simulink model "RoboBlock"  (R2020a)
settings: Solver=ode45  StartTime=0.0  StopTime=inf  FixedStep=0.050  RelTol=1e-3
model workspace (MAT data in the model file):
  Sig = Simulink.Signal
  Sig.DataType = 'auto'
  Sig.Dimensions = -1
  Sig.DimensionsMode = 'auto'
  Sig.Complexity = 'auto'
  Sig.SampleTime = -1
  Sig.SamplingMode = 'auto'
  Var = 0
libraries: simulink x2, dspmathops x1, fuzblock x1
settings Model: PauseTimes=7  Creator=user  LastModifiedBy=hjcam
settings DataIOCC: LimitDataPoints=on  SaveFormat=Array  ReturnWorkspaceOutputs=off
settings OptimizationCC: BlockReduction=off  BooleanDataType=off  LifeSpan=inf
settings DebuggingCC: SaveWithParameterizedLinksMsg=none  UnderspecifiedInitializationDetection=Classic  MergeDetectMultiDrivingBlocksExec=none  SignalResolutionControl=TryResolveAllWithWarning  SFUnexpectedBacktrackingDiag=warning  SFNoUnconditionalDefaultTransitionDiag=warning  SFExecutionAtInitializationDiag=none  ArithmeticOperatorsInVariantConditions=warning
settings HardwareCC: ProdBitPerPointer=32  ProdBitPerSizeT=32  ProdBitPerPtrDiffT=32  ProdLargestAtomicFloat=None  ProdIntDivRoundTo=Undefined  ProdEndianess=Unspecified  ProdWordSize=32  ProdHWDeviceType=32-bit Generic  TargetBitPerPointer=64  TargetBitPerSizeT=64  TargetBitPerPtrDiffT=64  TargetLongLongMode=on  TargetIntDivRoundTo=Zero  TargetEndianess=LittleEndian  TargetWordSize=64  TargetHWDeviceType=MATLAB Host  ProdEqTarget=off
settings ModelReferenceCC: PropagateSignalLabelsOutOfModel=off
settings SFSimCC: SimUseLocalCustomCode=off  CustomCodeUndefinedFunction=UseInterfaceOnly
settings RTWCC: RTWUseLocalCustomCode=off
settings CodeAppCC: StateflowObjectComments=on
settings GRTTargetCC: TargetLangStandard=C89/C90 (ANSI)
settings ConfigComp: CovMetricSettings=dw  CovHtmlReporting=on  CovSaveCumulativeToWorkspaceVar=on  CovSaveSingleToWorkspaceVar=on  CovExternalEMLEnable=off  CovSFcnEnable=off

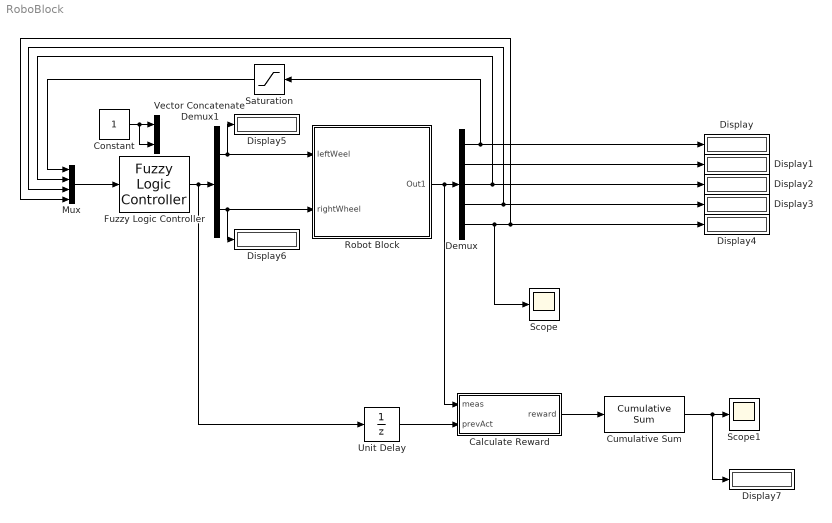
== system RoboBlock ==
  Calculate Reward : Subsystem
  Constant : Constant  VectorParams1D=off
  Cumulative Sum : dspmathops/Cumulative Sum  dim=Channels (running sum)  InputProcessing=Columns as channels (frame based)  reset_popup=None  roundingMode=Floor  overflowMode=off  outputDataTypeStr=Inherit: Same as accumulator  outputMin=[]  outputMax=[]  outputLastDataTypeStr=Inherit: Same as accumulator
  Demux : Demux  Outputs=5
  Demux1 : Demux  Outputs=2
  Display{,1..7} (8 alike) : Display
  Fuzzy Logic Controller : fuzblock/Fuzzy Logic  Controller  FIS=robot  OutputSampleNumber=101  DataType=double  FuzzifiedInputs=off  RuleFiringStrengths=off  RuleOutputs=off  AggregatedOutputs=off  SimulateUsing=Interpreted execution  OutOfRangeInputValueMessage=warning  NoRuleFiredMessage=warning  EmptyOutputFuzzySetMessage=warning
  Mux : Mux
  Robot Block : Subsystem  mask(Two-wheel Mobile Robot Model){stID=5013501, modeVal=off, initAngle=-0.628, simStep=0.050, Xpos=2.2597, Ypos=5.1629, isDemo=off}
      mask prompts: stID "Please Enter your UOW student number"; modeVal "Velocity Measurement Mode, select this to disable animations and to allow for the measurement of the velocity of the robot"; initAngle "Set the starting angle (Radians)"; simStep "Override Simulation Step (Defualt is 0.01)"; Xpos "(X,Y)"
      mask help:
      | Robot: Two-wheel robot is driven by two parallel wheels; the speed of each wheel could be set separately
      | Target: target is a single moving point in 2D space
      | Obstacle: obstacle is a group of polygons.
      | Block inputs:
      | vl : velocity of left wheel
      | vr : velocity of right wheel
      | Range of vl, vr: [-2, 2]
      | Block outputs:
      | theta: angle between robot facing and target bearing
      | dis: distance between robot and target
      | ob_loc
      | Range of obstacle detection sensor is 2.5
      | ob_loc=-9	No obstacle detected
      | ob_loc=-2.5	obstacle detected on the front left
      | ob_loc=-5	obstacle detected on the side left
      | ob_loc=0	obstacle detected in the middle
      | ob_loc=2.5	obstacle detected on the front right
      | ob_loc=5	obstacle detected on the side right
      | Battery level/Odometer: total remaining energy/Distance Travelled
      | ultrasonic: a logorithmic signal indicating the distance to the obstacle ( ie 0 = out of sight , a larger number = nearer to the obstacle )
      |
      | The system will crash if the robot collides with the obstacle.
      mask init:
      | stObj.stID = stID;
      | stObj.modeVal = modeVal;
      | stObj.simStep = simStep;
      | stObj.initPos = [Xpos Ypos initAngle];
      | stObj.isDemo = isDemo;
      mask Help:
      | Robot: Two-wheel robot is driven by two parallel wheels; the speed of each wheel could be set separately
      | Target: target is a single moving point in 2D space
      | Obstacle: obstacle is a group of polygons.
      | Block inputs:
      | vl : velocity of left wheel
      | vr : velocity of right wheel
      | Range of vl, vr: [-2, 2]
      | Block outputs:
      | theta: angle between robot facing and target bearing
      | dis: distance between robot and target
      | ob_loc
      | Range of obstacle detection sensor is 2.5
      | ob_loc=-9	No obstacle detected
      | ob_loc=-2.5	obstacle detected on the front left
      | ob_loc=-5	obstacle detected on the side left
      | ob_loc=0	obstacle detected in the middle
      | ob_loc=2.5	obstacle detected on the front right
      | ob_loc=5	obstacle detected on the side right
      | Battery level/Odometer: total remaining energy/Distance Travelled
      | ultrasonic: a logorithmic signal indicating the distance to the obstacle ( ie 0 = out of sight , a larger number = nearer to the obstacle )
      | 
      | The system will crash if the robot collides with the obstacle.
      mask Callback simStep:
      | pm = Simulink.Mask.get(gcb);
      | simStep = pm.getParameter('simStep');
      | set_param(gcs,'FixedStep', simStep.Value);
      mask DialogControl Container4 Prompt: Set the initial starting Coordinates and angle
      mask DialogControl Control3 Prompt: Set starting Position , (must be in the red shaded region)
      mask DialogControl Control3 Callback:
      | [out,~,~,~,~] = roboanimate_org([],[],[],'setup',[]);
      | Xpos = out(1);
      | Ypos = out(2);
      | p = Simulink.Mask.get(gcb);
      | p.Parameters(1,5).set('Value',num2str(Xpos));
      | p.Parameters(1,6).set('Value',num2str(Ypos));
      mask DialogControl Control5 Prompt: Initial Position:
      mask DialogControl Container4_copy Prompt: Run a demo
      mask DialogControl Control2 Prompt: Run  demo
      mask DialogControl Control2 Callback:
      | if(get_param(gcs,'SimulationStatus') == 'stopped')
      | 
      | pm = Simulink.Mask.get(gcb);
      | pm.Parameters(1,7).set('Value','on');
      | options = simset('SrcWorkspace','current');
      | try
      | sim(gcs,[],options)
      | pm.Parameters(1,7).set('Value','off');
      | catch
      | pm.Parameters(1,7).set('Value','off');
      | end
      | 
      | end
      mask Display:
      | patch([ -0.5 0.5 0.5 -0.5],[ -0.5 -0.5 0.5 0.5],[1 1 1])
      | 
      | patch([ -0.2 0.2 0.2 -0.2],[ -0.05 -0.05 0.05 0.05],[0 0 0])
      | 
      | patch(1.1*[ -0.15  0.15 0.15 -0.15],1.1*[ -0.15 -0.15 0.15 0.15],[0 0 0])
      | 
      | patch([ -0.15  0.15 0.15 -0.15],[ -0.15 -0.15 0.15 0.15],[0 0.8 0])
  Saturation : Saturate  UpperLimit=10
  Scope : Scope
  Scope1 : Scope
  Unit Delay : UnitDelay  SampleTime=-1  HasFrameUpgradeWarning=on
  Vector Concatenate : Concatenate
  wires:
  Robot Block/1(Out1) -> Calculate Reward/1(meas), Demux/1
  Demux/1 -> Saturation/1, Display/1
  Demux/2 -> Display1/1
  Demux/3 -> Mux/2, Display2/1
  Demux/5 -> Scope/1, Mux/4, Display4/1
  Demux1/2 -> Display6/1, Robot Block/2(rightWheel)
  Mux/1 -> Fuzzy Logic Controller/1
  Demux/4 -> Mux/3, Display3/1
  Saturation/1 -> Mux/1
  Demux1/1 -> Robot Block/1(leftWeel), Display5/1
  Unit Delay/1 -> Calculate Reward/2(prevAct)
  Calculate Reward/1(reward) -> Cumulative Sum/1
  Cumulative Sum/1 -> Display7/1, Scope1/1
  Constant/1 -> Vector Concatenate/2, Vector Concatenate/1
  Fuzzy Logic Controller/1 -> Unit Delay/1, Demux1/1

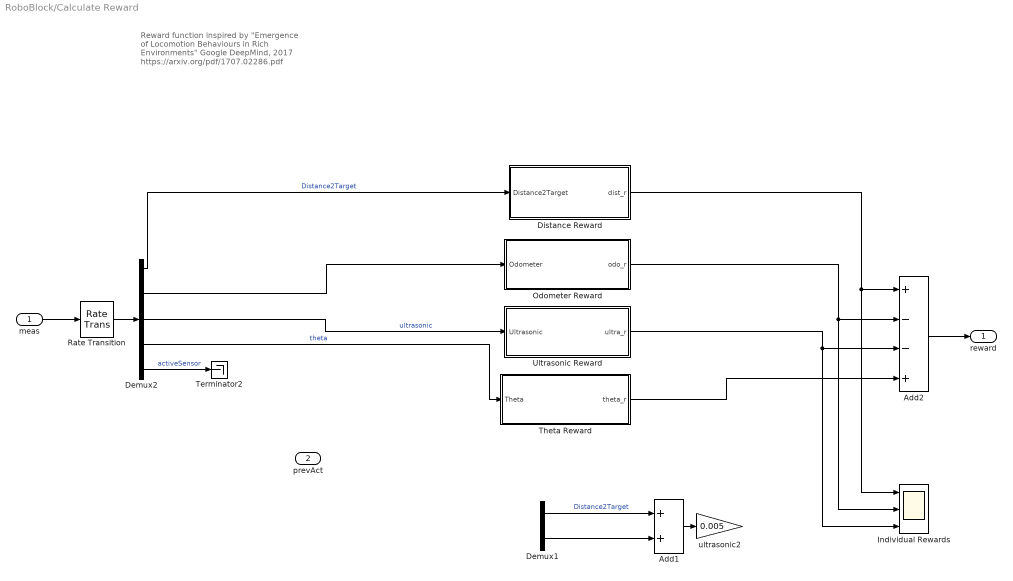
== system RoboBlock/Calculate Reward ==
  note: Reward function inspired by
      | "Emergence of Locomotion Behaviours in Rich Environments"
      | Google DeepMind, 2017
      | https://arxiv.org/pdf/1707.02286.pdf
  meas : Inport
  prevAct : Inport  Port=2
  Add1 : Sum
  Add2 : Sum  Inputs=+--+
  Demux1 : Demux  Outputs=2
  Demux2 : Demux  Outputs=5
  Distance Reward : Subsystem
  Individual Rewards : Scope  NumInputPorts=3
  Odometer Reward : Subsystem
  Rate Transition : RateTransition  OutPortSampleTime=Ts
  Terminator2 : Terminator
  Theta Reward : Subsystem
  Ultrasonic Reward : Subsystem
  ultrasonic2 : Gain  Gain=0.005
  reward : Outport  VectorParamsAs1DForOutWhenUnconnected=off
  wires:
  meas/1 -> Rate Transition/1
  Add2/1 -> reward/1
  Demux2/5 -> Terminator2/1  "activeSensor"
  Rate Transition/1 -> Demux2/1
  Demux2/4 -> Theta Reward/1(Theta)  "theta"
  Ultrasonic Reward/1(ultra_r) -> Individual Rewards/3, Add2/3
  Demux1/1 -> Add1/1  "Distance2Target"
  Demux1/2 -> Add1/2
  Add1/1 -> ultrasonic2/1
  Distance Reward/1(dist_r) -> Individual Rewards/1, Add2/1
  Demux2/1 -> Distance Reward/1(Distance2Target)  "Distance2Target"
  Odometer Reward/1(odo_r) -> Individual Rewards/2, Add2/2
  Demux2/2 -> Odometer Reward/1(Odometer)
  Demux2/3 -> Ultrasonic Reward/1(Ultrasonic)  "ultrasonic"
  Theta Reward/1(theta_r) -> Add2/4

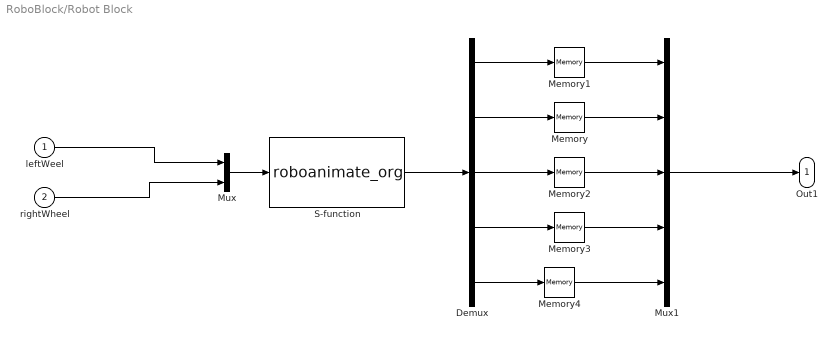
== system RoboBlock/Robot Block ==
  leftWeel : Inport
  rightWheel : Inport  Port=2
  Demux : Demux  Outputs=5
  Memory{,2..4} (4 alike) : Memory
  Memory1 : Memory  InitialCondition=1000
  Mux : Mux  Inputs=2
  Mux1 : Mux  Inputs=5
  S-function : S-Function  FunctionName=roboanimate_org  Parameters=stObj  SFunctionDeploymentMode=off  EnableBusSupport=off
  Out1 : Outport
  wires:
  rightWheel/1 -> Mux/2
  leftWeel/1 -> Mux/1
  Mux/1 -> S-function/1
  S-function/1 -> Demux/1
  Memory1/1 -> Mux1/1
  Demux/1 -> Memory1/1
  Memory/1 -> Mux1/2
  Memory2/1 -> Mux1/3
  Demux/3 -> Memory2/1
  Demux/2 -> Memory/1
  Demux/4 -> Memory3/1
  Memory3/1 -> Mux1/4
  Demux/5 -> Memory4/1
  Memory4/1 -> Mux1/5
  Mux1/1 -> Out1/1

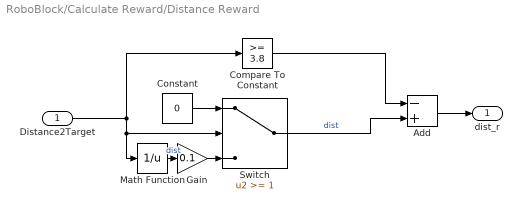
== system RoboBlock/Calculate Reward/Distance Reward ==
  Distance2Target : Inport
  Add : Sum  Inputs=-+
  Compare To Constant : simulink/Logic and Bit Operations/Compare To Constant  relop=>=  const=3.8  OutDataTypeStr=boolean
  Constant : Constant  Value=0
  Gain : Gain  Gain=0.1
  Math Function : Math  Operator=reciprocal  SaturateOnIntegerOverflow=on
  Switch : Switch  Threshold=1
  dist_r : Outport
  wires:
  Distance2Target/1 -> Switch/2, Math Function/1, Compare To Constant/1
  Switch/1 -> Add/2  "dist"
  Compare To Constant/1 -> Add/1
  Add/1 -> dist_r/1
  Constant/1 -> Switch/1
  Math Function/1 -> Gain/1  "dist"
  Gain/1 -> Switch/3

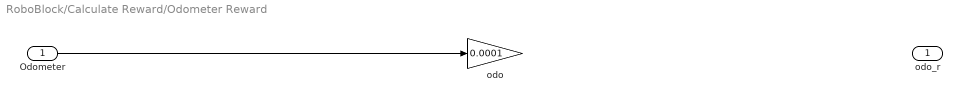
== system RoboBlock/Calculate Reward/Odometer Reward ==
  Odometer : Inport
  odo : Gain  Gain=0.0001
  odo_r : Outport
  wires:
  Odometer/1 -> odo/1

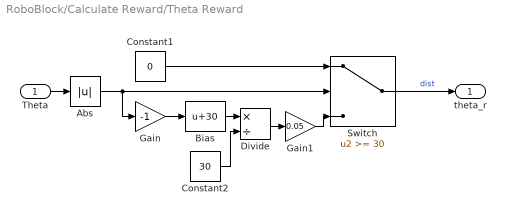
== system RoboBlock/Calculate Reward/Theta Reward ==
  Theta : Inport
  Abs : Abs
  Bias : Bias  Bias=30
  Constant1 : Constant  Value=0
  Constant2 : Constant  Value=30
  Divide : Product  Inputs=*/
  Gain : Gain  Gain=-1
  Gain1 : Gain  Gain=0.05
  Switch : Switch  Threshold=30
  theta_r : Outport
  wires:
  Theta/1 -> Abs/1
  Abs/1 -> Gain/1, Switch/2
  Constant1/1 -> Switch/1
  Gain/1 -> Bias/1
  Bias/1 -> Divide/1
  Constant2/1 -> Divide/2
  Divide/1 -> Gain1/1
  Gain1/1 -> Switch/3
  Switch/1 -> theta_r/1  "dist"

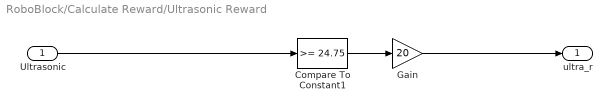
== system RoboBlock/Calculate Reward/Ultrasonic Reward ==
  Ultrasonic : Inport
  Compare To Constant1 : simulink/Logic and Bit Operations/Compare To Constant  relop=>=  const=24.75  OutDataTypeStr=boolean
  Gain : Gain  Gain=20
  ultra_r : Outport
  wires:
  Ultrasonic/1 -> Compare To Constant1/1
  Compare To Constant1/1 -> Gain/1
  Gain/1 -> ultra_r/1
